simulink model "gm_ZynqBF_2tx_fpga"  (R2018b)
settings: Solver=FixedStepDiscrete  StartTime=0.0  StopTime=10.0  FixedStep=(1/420e3)/128  RelTol=1e-3
undefined symbols (not defined in the file or in its folder): a, b, c
libraries: hdlsllib x873, simulink x349
(part 20 of 40)

== system gm_ZynqBF_2tx_fpga/channel_estimator/peakdetect_ch1/correlator1/rx_ram_q_instance39 ==
  i : Inport  OutDataTypeStr=fixdt(0, 6, 0)  PortDimensions=1  SampleTime=1.86011904761905e-08
  wdata : Inport  Port=2  OutDataTypeStr=fixdt(1, 16, 15)  PortDimensions=1  SampleTime=1.86011904761905e-08
  waddr : Inport  Port=3  OutDataTypeStr=fixdt(0, 9, 0)  PortDimensions=1  SampleTime=1.86011904761905e-08
  we : Inport  Port=4  OutDataTypeStr=fixdt(0, 64, 0)  PortDimensions=1  SampleTime=1.86011904761905e-08
  raddr : Inport  Port=5  OutDataTypeStr=fixdt(0, 10, 0)  PortDimensions=1  SampleTime=1.86011904761905e-08
  shift : Inport  Port=6  OutDataTypeStr=fixdt(0, 6, 0)  PortDimensions=1  SampleTime=1.86011904761905e-08
  Constant : Constant  OutDataTypeStr=fixdt(0, 1, 0)  SampleTime=-1
  Constant1 : Constant  OutDataTypeStr=fixdt(0, 1, 0)  SampleTime=-1
  Relational Operator : RelationalOperator  Operator=<  OutDataTypeStr=boolean  SampleTime=1.86011904761905e-08  RndMeth=Nearest
  Simple Dual Port RAM : hdlsllib/HDL RAMs/Simple Dual Port RAM  ram_size=9
      settings: SourceProductName=HDL Coder  SourceProductBaseCode=HD
  Sum : Sum  AccumDataTypeStr=fixdt(0, 11, 0)  OutDataTypeStr=fixdt(0, 9, 0)  SampleTime=1.86011904761905e-08
  Sum1 : Sum  AccumDataTypeStr=fixdt(0, 7, 0)  OutDataTypeStr=fixdt(0, 9, 0)  SampleTime=1.86011904761905e-08
  Switch : Switch  Criteria=u2 ~= 0  Threshold=double(0)  OutDataTypeStr=fixdt(0, 9, 0)  SampleTime=1.86011904761905e-08
  get_bit : Subsystem
  dout : Outport
  probe : Outport  Port=2
  wires:
  shift/1 -> Relational Operator/2
  raddr/1 -> Switch/3, Sum/2
  we/1 -> get_bit/1(u)
  waddr/1 -> Simple Dual Port RAM/2
  wdata/1 -> Simple Dual Port RAM/1
  i/1 -> Sum1/1, Relational Operator/1
  Constant/1 -> Sum/1
  Constant1/1 -> Sum1/2
  Relational Operator/1 -> Switch/2
  Simple Dual Port RAM/1 -> dout/1
  Sum/1 -> Switch/1
  Sum1/1 -> get_bit/2(ind)
  Switch/1 -> Simple Dual Port RAM/4, probe/1
  get_bit/1(y) -> Simple Dual Port RAM/3

== system gm_ZynqBF_2tx_fpga/channel_estimator/peakdetect_ch1/correlator1/rx_ram_q_instance4 ==
  i : Inport  OutDataTypeStr=fixdt(0, 6, 0)  PortDimensions=1  SampleTime=1.86011904761905e-08
  wdata : Inport  Port=2  OutDataTypeStr=fixdt(1, 16, 15)  PortDimensions=1  SampleTime=1.86011904761905e-08
  waddr : Inport  Port=3  OutDataTypeStr=fixdt(0, 9, 0)  PortDimensions=1  SampleTime=1.86011904761905e-08
  we : Inport  Port=4  OutDataTypeStr=fixdt(0, 64, 0)  PortDimensions=1  SampleTime=1.86011904761905e-08
  raddr : Inport  Port=5  OutDataTypeStr=fixdt(0, 10, 0)  PortDimensions=1  SampleTime=1.86011904761905e-08
  shift : Inport  Port=6  OutDataTypeStr=fixdt(0, 6, 0)  PortDimensions=1  SampleTime=1.86011904761905e-08
  Constant : Constant  OutDataTypeStr=fixdt(0, 1, 0)  SampleTime=-1
  Constant1 : Constant  OutDataTypeStr=fixdt(0, 1, 0)  SampleTime=-1
  Relational Operator : RelationalOperator  Operator=<  OutDataTypeStr=boolean  SampleTime=1.86011904761905e-08  RndMeth=Nearest
  Simple Dual Port RAM : hdlsllib/HDL RAMs/Simple Dual Port RAM  ram_size=9
      settings: SourceProductName=HDL Coder  SourceProductBaseCode=HD
  Sum : Sum  AccumDataTypeStr=fixdt(0, 11, 0)  OutDataTypeStr=fixdt(0, 9, 0)  SampleTime=1.86011904761905e-08
  Sum1 : Sum  AccumDataTypeStr=fixdt(0, 7, 0)  OutDataTypeStr=fixdt(0, 9, 0)  SampleTime=1.86011904761905e-08
  Switch : Switch  Criteria=u2 ~= 0  Threshold=double(0)  OutDataTypeStr=fixdt(0, 9, 0)  SampleTime=1.86011904761905e-08
  get_bit : Subsystem
  dout : Outport
  probe : Outport  Port=2
  wires:
  shift/1 -> Relational Operator/2
  raddr/1 -> Switch/3, Sum/2
  we/1 -> get_bit/1(u)
  waddr/1 -> Simple Dual Port RAM/2
  wdata/1 -> Simple Dual Port RAM/1
  i/1 -> Sum1/1, Relational Operator/1
  Constant/1 -> Sum/1
  Constant1/1 -> Sum1/2
  Relational Operator/1 -> Switch/2
  Simple Dual Port RAM/1 -> dout/1
  Sum/1 -> Switch/1
  Sum1/1 -> get_bit/2(ind)
  Switch/1 -> Simple Dual Port RAM/4, probe/1
  get_bit/1(y) -> Simple Dual Port RAM/3

== system gm_ZynqBF_2tx_fpga/channel_estimator/peakdetect_ch1/correlator1/rx_ram_q_instance40 ==
  i : Inport  OutDataTypeStr=fixdt(0, 6, 0)  PortDimensions=1  SampleTime=1.86011904761905e-08
  wdata : Inport  Port=2  OutDataTypeStr=fixdt(1, 16, 15)  PortDimensions=1  SampleTime=1.86011904761905e-08
  waddr : Inport  Port=3  OutDataTypeStr=fixdt(0, 9, 0)  PortDimensions=1  SampleTime=1.86011904761905e-08
  we : Inport  Port=4  OutDataTypeStr=fixdt(0, 64, 0)  PortDimensions=1  SampleTime=1.86011904761905e-08
  raddr : Inport  Port=5  OutDataTypeStr=fixdt(0, 10, 0)  PortDimensions=1  SampleTime=1.86011904761905e-08
  shift : Inport  Port=6  OutDataTypeStr=fixdt(0, 6, 0)  PortDimensions=1  SampleTime=1.86011904761905e-08
  Constant : Constant  OutDataTypeStr=fixdt(0, 1, 0)  SampleTime=-1
  Constant1 : Constant  OutDataTypeStr=fixdt(0, 1, 0)  SampleTime=-1
  Relational Operator : RelationalOperator  Operator=<  OutDataTypeStr=boolean  SampleTime=1.86011904761905e-08  RndMeth=Nearest
  Simple Dual Port RAM : hdlsllib/HDL RAMs/Simple Dual Port RAM  ram_size=9
      settings: SourceProductName=HDL Coder  SourceProductBaseCode=HD
  Sum : Sum  AccumDataTypeStr=fixdt(0, 11, 0)  OutDataTypeStr=fixdt(0, 9, 0)  SampleTime=1.86011904761905e-08
  Sum1 : Sum  AccumDataTypeStr=fixdt(0, 7, 0)  OutDataTypeStr=fixdt(0, 9, 0)  SampleTime=1.86011904761905e-08
  Switch : Switch  Criteria=u2 ~= 0  Threshold=double(0)  OutDataTypeStr=fixdt(0, 9, 0)  SampleTime=1.86011904761905e-08
  get_bit : Subsystem
  dout : Outport
  probe : Outport  Port=2
  wires:
  shift/1 -> Relational Operator/2
  raddr/1 -> Switch/3, Sum/2
  we/1 -> get_bit/1(u)
  waddr/1 -> Simple Dual Port RAM/2
  wdata/1 -> Simple Dual Port RAM/1
  i/1 -> Sum1/1, Relational Operator/1
  Constant/1 -> Sum/1
  Constant1/1 -> Sum1/2
  Relational Operator/1 -> Switch/2
  Simple Dual Port RAM/1 -> dout/1
  Sum/1 -> Switch/1
  Sum1/1 -> get_bit/2(ind)
  Switch/1 -> Simple Dual Port RAM/4, probe/1
  get_bit/1(y) -> Simple Dual Port RAM/3

== system gm_ZynqBF_2tx_fpga/channel_estimator/peakdetect_ch1/correlator1/rx_ram_q_instance41 ==
  i : Inport  OutDataTypeStr=fixdt(0, 6, 0)  PortDimensions=1  SampleTime=1.86011904761905e-08
  wdata : Inport  Port=2  OutDataTypeStr=fixdt(1, 16, 15)  PortDimensions=1  SampleTime=1.86011904761905e-08
  waddr : Inport  Port=3  OutDataTypeStr=fixdt(0, 9, 0)  PortDimensions=1  SampleTime=1.86011904761905e-08
  we : Inport  Port=4  OutDataTypeStr=fixdt(0, 64, 0)  PortDimensions=1  SampleTime=1.86011904761905e-08
  raddr : Inport  Port=5  OutDataTypeStr=fixdt(0, 10, 0)  PortDimensions=1  SampleTime=1.86011904761905e-08
  shift : Inport  Port=6  OutDataTypeStr=fixdt(0, 6, 0)  PortDimensions=1  SampleTime=1.86011904761905e-08
  Constant : Constant  OutDataTypeStr=fixdt(0, 1, 0)  SampleTime=-1
  Constant1 : Constant  OutDataTypeStr=fixdt(0, 1, 0)  SampleTime=-1
  Relational Operator : RelationalOperator  Operator=<  OutDataTypeStr=boolean  SampleTime=1.86011904761905e-08  RndMeth=Nearest
  Simple Dual Port RAM : hdlsllib/HDL RAMs/Simple Dual Port RAM  ram_size=9
      settings: SourceProductName=HDL Coder  SourceProductBaseCode=HD
  Sum : Sum  AccumDataTypeStr=fixdt(0, 11, 0)  OutDataTypeStr=fixdt(0, 9, 0)  SampleTime=1.86011904761905e-08
  Sum1 : Sum  AccumDataTypeStr=fixdt(0, 7, 0)  OutDataTypeStr=fixdt(0, 9, 0)  SampleTime=1.86011904761905e-08
  Switch : Switch  Criteria=u2 ~= 0  Threshold=double(0)  OutDataTypeStr=fixdt(0, 9, 0)  SampleTime=1.86011904761905e-08
  get_bit : Subsystem
  dout : Outport
  probe : Outport  Port=2
  wires:
  shift/1 -> Relational Operator/2
  raddr/1 -> Switch/3, Sum/2
  we/1 -> get_bit/1(u)
  waddr/1 -> Simple Dual Port RAM/2
  wdata/1 -> Simple Dual Port RAM/1
  i/1 -> Sum1/1, Relational Operator/1
  Constant/1 -> Sum/1
  Constant1/1 -> Sum1/2
  Relational Operator/1 -> Switch/2
  Simple Dual Port RAM/1 -> dout/1
  Sum/1 -> Switch/1
  Sum1/1 -> get_bit/2(ind)
  Switch/1 -> Simple Dual Port RAM/4, probe/1
  get_bit/1(y) -> Simple Dual Port RAM/3

== system gm_ZynqBF_2tx_fpga/channel_estimator/peakdetect_ch1/correlator1/rx_ram_q_instance42 ==
  i : Inport  OutDataTypeStr=fixdt(0, 6, 0)  PortDimensions=1  SampleTime=1.86011904761905e-08
  wdata : Inport  Port=2  OutDataTypeStr=fixdt(1, 16, 15)  PortDimensions=1  SampleTime=1.86011904761905e-08
  waddr : Inport  Port=3  OutDataTypeStr=fixdt(0, 9, 0)  PortDimensions=1  SampleTime=1.86011904761905e-08
  we : Inport  Port=4  OutDataTypeStr=fixdt(0, 64, 0)  PortDimensions=1  SampleTime=1.86011904761905e-08
  raddr : Inport  Port=5  OutDataTypeStr=fixdt(0, 10, 0)  PortDimensions=1  SampleTime=1.86011904761905e-08
  shift : Inport  Port=6  OutDataTypeStr=fixdt(0, 6, 0)  PortDimensions=1  SampleTime=1.86011904761905e-08
  Constant : Constant  OutDataTypeStr=fixdt(0, 1, 0)  SampleTime=-1
  Constant1 : Constant  OutDataTypeStr=fixdt(0, 1, 0)  SampleTime=-1
  Relational Operator : RelationalOperator  Operator=<  OutDataTypeStr=boolean  SampleTime=1.86011904761905e-08  RndMeth=Nearest
  Simple Dual Port RAM : hdlsllib/HDL RAMs/Simple Dual Port RAM  ram_size=9
      settings: SourceProductName=HDL Coder  SourceProductBaseCode=HD
  Sum : Sum  AccumDataTypeStr=fixdt(0, 11, 0)  OutDataTypeStr=fixdt(0, 9, 0)  SampleTime=1.86011904761905e-08
  Sum1 : Sum  AccumDataTypeStr=fixdt(0, 7, 0)  OutDataTypeStr=fixdt(0, 9, 0)  SampleTime=1.86011904761905e-08
  Switch : Switch  Criteria=u2 ~= 0  Threshold=double(0)  OutDataTypeStr=fixdt(0, 9, 0)  SampleTime=1.86011904761905e-08
  get_bit : Subsystem
  dout : Outport
  probe : Outport  Port=2
  wires:
  shift/1 -> Relational Operator/2
  raddr/1 -> Switch/3, Sum/2
  we/1 -> get_bit/1(u)
  waddr/1 -> Simple Dual Port RAM/2
  wdata/1 -> Simple Dual Port RAM/1
  i/1 -> Sum1/1, Relational Operator/1
  Constant/1 -> Sum/1
  Constant1/1 -> Sum1/2
  Relational Operator/1 -> Switch/2
  Simple Dual Port RAM/1 -> dout/1
  Sum/1 -> Switch/1
  Sum1/1 -> get_bit/2(ind)
  Switch/1 -> Simple Dual Port RAM/4, probe/1
  get_bit/1(y) -> Simple Dual Port RAM/3

== system gm_ZynqBF_2tx_fpga/channel_estimator/peakdetect_ch1/correlator1/rx_ram_q_instance43 ==
  i : Inport  OutDataTypeStr=fixdt(0, 6, 0)  PortDimensions=1  SampleTime=1.86011904761905e-08
  wdata : Inport  Port=2  OutDataTypeStr=fixdt(1, 16, 15)  PortDimensions=1  SampleTime=1.86011904761905e-08
  waddr : Inport  Port=3  OutDataTypeStr=fixdt(0, 9, 0)  PortDimensions=1  SampleTime=1.86011904761905e-08
  we : Inport  Port=4  OutDataTypeStr=fixdt(0, 64, 0)  PortDimensions=1  SampleTime=1.86011904761905e-08
  raddr : Inport  Port=5  OutDataTypeStr=fixdt(0, 10, 0)  PortDimensions=1  SampleTime=1.86011904761905e-08
  shift : Inport  Port=6  OutDataTypeStr=fixdt(0, 6, 0)  PortDimensions=1  SampleTime=1.86011904761905e-08
  Constant : Constant  OutDataTypeStr=fixdt(0, 1, 0)  SampleTime=-1
  Constant1 : Constant  OutDataTypeStr=fixdt(0, 1, 0)  SampleTime=-1
  Relational Operator : RelationalOperator  Operator=<  OutDataTypeStr=boolean  SampleTime=1.86011904761905e-08  RndMeth=Nearest
  Simple Dual Port RAM : hdlsllib/HDL RAMs/Simple Dual Port RAM  ram_size=9
      settings: SourceProductName=HDL Coder  SourceProductBaseCode=HD
  Sum : Sum  AccumDataTypeStr=fixdt(0, 11, 0)  OutDataTypeStr=fixdt(0, 9, 0)  SampleTime=1.86011904761905e-08
  Sum1 : Sum  AccumDataTypeStr=fixdt(0, 7, 0)  OutDataTypeStr=fixdt(0, 9, 0)  SampleTime=1.86011904761905e-08
  Switch : Switch  Criteria=u2 ~= 0  Threshold=double(0)  OutDataTypeStr=fixdt(0, 9, 0)  SampleTime=1.86011904761905e-08
  get_bit : Subsystem
  dout : Outport
  probe : Outport  Port=2
  wires:
  shift/1 -> Relational Operator/2
  raddr/1 -> Switch/3, Sum/2
  we/1 -> get_bit/1(u)
  waddr/1 -> Simple Dual Port RAM/2
  wdata/1 -> Simple Dual Port RAM/1
  i/1 -> Sum1/1, Relational Operator/1
  Constant/1 -> Sum/1
  Constant1/1 -> Sum1/2
  Relational Operator/1 -> Switch/2
  Simple Dual Port RAM/1 -> dout/1
  Sum/1 -> Switch/1
  Sum1/1 -> get_bit/2(ind)
  Switch/1 -> Simple Dual Port RAM/4, probe/1
  get_bit/1(y) -> Simple Dual Port RAM/3

== system gm_ZynqBF_2tx_fpga/channel_estimator/peakdetect_ch1/correlator1/rx_ram_q_instance44 ==
  i : Inport  OutDataTypeStr=fixdt(0, 6, 0)  PortDimensions=1  SampleTime=1.86011904761905e-08
  wdata : Inport  Port=2  OutDataTypeStr=fixdt(1, 16, 15)  PortDimensions=1  SampleTime=1.86011904761905e-08
  waddr : Inport  Port=3  OutDataTypeStr=fixdt(0, 9, 0)  PortDimensions=1  SampleTime=1.86011904761905e-08
  we : Inport  Port=4  OutDataTypeStr=fixdt(0, 64, 0)  PortDimensions=1  SampleTime=1.86011904761905e-08
  raddr : Inport  Port=5  OutDataTypeStr=fixdt(0, 10, 0)  PortDimensions=1  SampleTime=1.86011904761905e-08
  shift : Inport  Port=6  OutDataTypeStr=fixdt(0, 6, 0)  PortDimensions=1  SampleTime=1.86011904761905e-08
  Constant : Constant  OutDataTypeStr=fixdt(0, 1, 0)  SampleTime=-1
  Constant1 : Constant  OutDataTypeStr=fixdt(0, 1, 0)  SampleTime=-1
  Relational Operator : RelationalOperator  Operator=<  OutDataTypeStr=boolean  SampleTime=1.86011904761905e-08  RndMeth=Nearest
  Simple Dual Port RAM : hdlsllib/HDL RAMs/Simple Dual Port RAM  ram_size=9
      settings: SourceProductName=HDL Coder  SourceProductBaseCode=HD
  Sum : Sum  AccumDataTypeStr=fixdt(0, 11, 0)  OutDataTypeStr=fixdt(0, 9, 0)  SampleTime=1.86011904761905e-08
  Sum1 : Sum  AccumDataTypeStr=fixdt(0, 7, 0)  OutDataTypeStr=fixdt(0, 9, 0)  SampleTime=1.86011904761905e-08
  Switch : Switch  Criteria=u2 ~= 0  Threshold=double(0)  OutDataTypeStr=fixdt(0, 9, 0)  SampleTime=1.86011904761905e-08
  get_bit : Subsystem
  dout : Outport
  probe : Outport  Port=2
  wires:
  shift/1 -> Relational Operator/2
  raddr/1 -> Switch/3, Sum/2
  we/1 -> get_bit/1(u)
  waddr/1 -> Simple Dual Port RAM/2
  wdata/1 -> Simple Dual Port RAM/1
  i/1 -> Sum1/1, Relational Operator/1
  Constant/1 -> Sum/1
  Constant1/1 -> Sum1/2
  Relational Operator/1 -> Switch/2
  Simple Dual Port RAM/1 -> dout/1
  Sum/1 -> Switch/1
  Sum1/1 -> get_bit/2(ind)
  Switch/1 -> Simple Dual Port RAM/4, probe/1
  get_bit/1(y) -> Simple Dual Port RAM/3

== system gm_ZynqBF_2tx_fpga/channel_estimator/peakdetect_ch1/correlator1/rx_ram_q_instance45 ==
  i : Inport  OutDataTypeStr=fixdt(0, 6, 0)  PortDimensions=1  SampleTime=1.86011904761905e-08
  wdata : Inport  Port=2  OutDataTypeStr=fixdt(1, 16, 15)  PortDimensions=1  SampleTime=1.86011904761905e-08
  waddr : Inport  Port=3  OutDataTypeStr=fixdt(0, 9, 0)  PortDimensions=1  SampleTime=1.86011904761905e-08
  we : Inport  Port=4  OutDataTypeStr=fixdt(0, 64, 0)  PortDimensions=1  SampleTime=1.86011904761905e-08
  raddr : Inport  Port=5  OutDataTypeStr=fixdt(0, 10, 0)  PortDimensions=1  SampleTime=1.86011904761905e-08
  shift : Inport  Port=6  OutDataTypeStr=fixdt(0, 6, 0)  PortDimensions=1  SampleTime=1.86011904761905e-08
  Constant : Constant  OutDataTypeStr=fixdt(0, 1, 0)  SampleTime=-1
  Constant1 : Constant  OutDataTypeStr=fixdt(0, 1, 0)  SampleTime=-1
  Relational Operator : RelationalOperator  Operator=<  OutDataTypeStr=boolean  SampleTime=1.86011904761905e-08  RndMeth=Nearest
  Simple Dual Port RAM : hdlsllib/HDL RAMs/Simple Dual Port RAM  ram_size=9
      settings: SourceProductName=HDL Coder  SourceProductBaseCode=HD
  Sum : Sum  AccumDataTypeStr=fixdt(0, 11, 0)  OutDataTypeStr=fixdt(0, 9, 0)  SampleTime=1.86011904761905e-08
  Sum1 : Sum  AccumDataTypeStr=fixdt(0, 7, 0)  OutDataTypeStr=fixdt(0, 9, 0)  SampleTime=1.86011904761905e-08
  Switch : Switch  Criteria=u2 ~= 0  Threshold=double(0)  OutDataTypeStr=fixdt(0, 9, 0)  SampleTime=1.86011904761905e-08
  get_bit : Subsystem
  dout : Outport
  probe : Outport  Port=2
  wires:
  shift/1 -> Relational Operator/2
  raddr/1 -> Switch/3, Sum/2
  we/1 -> get_bit/1(u)
  waddr/1 -> Simple Dual Port RAM/2
  wdata/1 -> Simple Dual Port RAM/1
  i/1 -> Sum1/1, Relational Operator/1
  Constant/1 -> Sum/1
  Constant1/1 -> Sum1/2
  Relational Operator/1 -> Switch/2
  Simple Dual Port RAM/1 -> dout/1
  Sum/1 -> Switch/1
  Sum1/1 -> get_bit/2(ind)
  Switch/1 -> Simple Dual Port RAM/4, probe/1
  get_bit/1(y) -> Simple Dual Port RAM/3

== system gm_ZynqBF_2tx_fpga/channel_estimator/peakdetect_ch1/correlator1/rx_ram_q_instance46 ==
  i : Inport  OutDataTypeStr=fixdt(0, 6, 0)  PortDimensions=1  SampleTime=1.86011904761905e-08
  wdata : Inport  Port=2  OutDataTypeStr=fixdt(1, 16, 15)  PortDimensions=1  SampleTime=1.86011904761905e-08
  waddr : Inport  Port=3  OutDataTypeStr=fixdt(0, 9, 0)  PortDimensions=1  SampleTime=1.86011904761905e-08
  we : Inport  Port=4  OutDataTypeStr=fixdt(0, 64, 0)  PortDimensions=1  SampleTime=1.86011904761905e-08
  raddr : Inport  Port=5  OutDataTypeStr=fixdt(0, 10, 0)  PortDimensions=1  SampleTime=1.86011904761905e-08
  shift : Inport  Port=6  OutDataTypeStr=fixdt(0, 6, 0)  PortDimensions=1  SampleTime=1.86011904761905e-08
  Constant : Constant  OutDataTypeStr=fixdt(0, 1, 0)  SampleTime=-1
  Constant1 : Constant  OutDataTypeStr=fixdt(0, 1, 0)  SampleTime=-1
  Relational Operator : RelationalOperator  Operator=<  OutDataTypeStr=boolean  SampleTime=1.86011904761905e-08  RndMeth=Nearest
  Simple Dual Port RAM : hdlsllib/HDL RAMs/Simple Dual Port RAM  ram_size=9
      settings: SourceProductName=HDL Coder  SourceProductBaseCode=HD
  Sum : Sum  AccumDataTypeStr=fixdt(0, 11, 0)  OutDataTypeStr=fixdt(0, 9, 0)  SampleTime=1.86011904761905e-08
  Sum1 : Sum  AccumDataTypeStr=fixdt(0, 7, 0)  OutDataTypeStr=fixdt(0, 9, 0)  SampleTime=1.86011904761905e-08
  Switch : Switch  Criteria=u2 ~= 0  Threshold=double(0)  OutDataTypeStr=fixdt(0, 9, 0)  SampleTime=1.86011904761905e-08
  get_bit : Subsystem
  dout : Outport
  probe : Outport  Port=2
  wires:
  shift/1 -> Relational Operator/2
  raddr/1 -> Switch/3, Sum/2
  we/1 -> get_bit/1(u)
  waddr/1 -> Simple Dual Port RAM/2
  wdata/1 -> Simple Dual Port RAM/1
  i/1 -> Sum1/1, Relational Operator/1
  Constant/1 -> Sum/1
  Constant1/1 -> Sum1/2
  Relational Operator/1 -> Switch/2
  Simple Dual Port RAM/1 -> dout/1
  Sum/1 -> Switch/1
  Sum1/1 -> get_bit/2(ind)
  Switch/1 -> Simple Dual Port RAM/4, probe/1
  get_bit/1(y) -> Simple Dual Port RAM/3

== system gm_ZynqBF_2tx_fpga/channel_estimator/peakdetect_ch1/correlator1/rx_ram_q_instance47 ==
  i : Inport  OutDataTypeStr=fixdt(0, 6, 0)  PortDimensions=1  SampleTime=1.86011904761905e-08
  wdata : Inport  Port=2  OutDataTypeStr=fixdt(1, 16, 15)  PortDimensions=1  SampleTime=1.86011904761905e-08
  waddr : Inport  Port=3  OutDataTypeStr=fixdt(0, 9, 0)  PortDimensions=1  SampleTime=1.86011904761905e-08
  we : Inport  Port=4  OutDataTypeStr=fixdt(0, 64, 0)  PortDimensions=1  SampleTime=1.86011904761905e-08
  raddr : Inport  Port=5  OutDataTypeStr=fixdt(0, 10, 0)  PortDimensions=1  SampleTime=1.86011904761905e-08
  shift : Inport  Port=6  OutDataTypeStr=fixdt(0, 6, 0)  PortDimensions=1  SampleTime=1.86011904761905e-08
  Constant : Constant  OutDataTypeStr=fixdt(0, 1, 0)  SampleTime=-1
  Constant1 : Constant  OutDataTypeStr=fixdt(0, 1, 0)  SampleTime=-1
  Relational Operator : RelationalOperator  Operator=<  OutDataTypeStr=boolean  SampleTime=1.86011904761905e-08  RndMeth=Nearest
  Simple Dual Port RAM : hdlsllib/HDL RAMs/Simple Dual Port RAM  ram_size=9
      settings: SourceProductName=HDL Coder  SourceProductBaseCode=HD
  Sum : Sum  AccumDataTypeStr=fixdt(0, 11, 0)  OutDataTypeStr=fixdt(0, 9, 0)  SampleTime=1.86011904761905e-08
  Sum1 : Sum  AccumDataTypeStr=fixdt(0, 7, 0)  OutDataTypeStr=fixdt(0, 9, 0)  SampleTime=1.86011904761905e-08
  Switch : Switch  Criteria=u2 ~= 0  Threshold=double(0)  OutDataTypeStr=fixdt(0, 9, 0)  SampleTime=1.86011904761905e-08
  get_bit : Subsystem
  dout : Outport
  probe : Outport  Port=2
  wires:
  shift/1 -> Relational Operator/2
  raddr/1 -> Switch/3, Sum/2
  we/1 -> get_bit/1(u)
  waddr/1 -> Simple Dual Port RAM/2
  wdata/1 -> Simple Dual Port RAM/1
  i/1 -> Sum1/1, Relational Operator/1
  Constant/1 -> Sum/1
  Constant1/1 -> Sum1/2
  Relational Operator/1 -> Switch/2
  Simple Dual Port RAM/1 -> dout/1
  Sum/1 -> Switch/1
  Sum1/1 -> get_bit/2(ind)
  Switch/1 -> Simple Dual Port RAM/4, probe/1
  get_bit/1(y) -> Simple Dual Port RAM/3

== system gm_ZynqBF_2tx_fpga/channel_estimator/peakdetect_ch1/correlator1/rx_ram_q_instance48 ==
  i : Inport  OutDataTypeStr=fixdt(0, 6, 0)  PortDimensions=1  SampleTime=1.86011904761905e-08
  wdata : Inport  Port=2  OutDataTypeStr=fixdt(1, 16, 15)  PortDimensions=1  SampleTime=1.86011904761905e-08
  waddr : Inport  Port=3  OutDataTypeStr=fixdt(0, 9, 0)  PortDimensions=1  SampleTime=1.86011904761905e-08
  we : Inport  Port=4  OutDataTypeStr=fixdt(0, 64, 0)  PortDimensions=1  SampleTime=1.86011904761905e-08
  raddr : Inport  Port=5  OutDataTypeStr=fixdt(0, 10, 0)  PortDimensions=1  SampleTime=1.86011904761905e-08
  shift : Inport  Port=6  OutDataTypeStr=fixdt(0, 6, 0)  PortDimensions=1  SampleTime=1.86011904761905e-08
  Constant : Constant  OutDataTypeStr=fixdt(0, 1, 0)  SampleTime=-1
  Constant1 : Constant  OutDataTypeStr=fixdt(0, 1, 0)  SampleTime=-1
  Relational Operator : RelationalOperator  Operator=<  OutDataTypeStr=boolean  SampleTime=1.86011904761905e-08  RndMeth=Nearest
  Simple Dual Port RAM : hdlsllib/HDL RAMs/Simple Dual Port RAM  ram_size=9
      settings: SourceProductName=HDL Coder  SourceProductBaseCode=HD
  Sum : Sum  AccumDataTypeStr=fixdt(0, 11, 0)  OutDataTypeStr=fixdt(0, 9, 0)  SampleTime=1.86011904761905e-08
  Sum1 : Sum  AccumDataTypeStr=fixdt(0, 7, 0)  OutDataTypeStr=fixdt(0, 9, 0)  SampleTime=1.86011904761905e-08
  Switch : Switch  Criteria=u2 ~= 0  Threshold=double(0)  OutDataTypeStr=fixdt(0, 9, 0)  SampleTime=1.86011904761905e-08
  get_bit : Subsystem
  dout : Outport
  probe : Outport  Port=2
  wires:
  shift/1 -> Relational Operator/2
  raddr/1 -> Switch/3, Sum/2
  we/1 -> get_bit/1(u)
  waddr/1 -> Simple Dual Port RAM/2
  wdata/1 -> Simple Dual Port RAM/1
  i/1 -> Sum1/1, Relational Operator/1
  Constant/1 -> Sum/1
  Constant1/1 -> Sum1/2
  Relational Operator/1 -> Switch/2
  Simple Dual Port RAM/1 -> dout/1
  Sum/1 -> Switch/1
  Sum1/1 -> get_bit/2(ind)
  Switch/1 -> Simple Dual Port RAM/4, probe/1
  get_bit/1(y) -> Simple Dual Port RAM/3

== system gm_ZynqBF_2tx_fpga/channel_estimator/peakdetect_ch1/correlator1/rx_ram_q_instance49 ==
  i : Inport  OutDataTypeStr=fixdt(0, 6, 0)  PortDimensions=1  SampleTime=1.86011904761905e-08
  wdata : Inport  Port=2  OutDataTypeStr=fixdt(1, 16, 15)  PortDimensions=1  SampleTime=1.86011904761905e-08
  waddr : Inport  Port=3  OutDataTypeStr=fixdt(0, 9, 0)  PortDimensions=1  SampleTime=1.86011904761905e-08
  we : Inport  Port=4  OutDataTypeStr=fixdt(0, 64, 0)  PortDimensions=1  SampleTime=1.86011904761905e-08
  raddr : Inport  Port=5  OutDataTypeStr=fixdt(0, 10, 0)  PortDimensions=1  SampleTime=1.86011904761905e-08
  shift : Inport  Port=6  OutDataTypeStr=fixdt(0, 6, 0)  PortDimensions=1  SampleTime=1.86011904761905e-08
  Constant : Constant  OutDataTypeStr=fixdt(0, 1, 0)  SampleTime=-1
  Constant1 : Constant  OutDataTypeStr=fixdt(0, 1, 0)  SampleTime=-1
  Relational Operator : RelationalOperator  Operator=<  OutDataTypeStr=boolean  SampleTime=1.86011904761905e-08  RndMeth=Nearest
  Simple Dual Port RAM : hdlsllib/HDL RAMs/Simple Dual Port RAM  ram_size=9
      settings: SourceProductName=HDL Coder  SourceProductBaseCode=HD
  Sum : Sum  AccumDataTypeStr=fixdt(0, 11, 0)  OutDataTypeStr=fixdt(0, 9, 0)  SampleTime=1.86011904761905e-08
  Sum1 : Sum  AccumDataTypeStr=fixdt(0, 7, 0)  OutDataTypeStr=fixdt(0, 9, 0)  SampleTime=1.86011904761905e-08
  Switch : Switch  Criteria=u2 ~= 0  Threshold=double(0)  OutDataTypeStr=fixdt(0, 9, 0)  SampleTime=1.86011904761905e-08
  get_bit : Subsystem
  dout : Outport
  probe : Outport  Port=2
  wires:
  shift/1 -> Relational Operator/2
  raddr/1 -> Switch/3, Sum/2
  we/1 -> get_bit/1(u)
  waddr/1 -> Simple Dual Port RAM/2
  wdata/1 -> Simple Dual Port RAM/1
  i/1 -> Sum1/1, Relational Operator/1
  Constant/1 -> Sum/1
  Constant1/1 -> Sum1/2
  Relational Operator/1 -> Switch/2
  Simple Dual Port RAM/1 -> dout/1
  Sum/1 -> Switch/1
  Sum1/1 -> get_bit/2(ind)
  Switch/1 -> Simple Dual Port RAM/4, probe/1
  get_bit/1(y) -> Simple Dual Port RAM/3

== system gm_ZynqBF_2tx_fpga/channel_estimator/peakdetect_ch1/correlator1/rx_ram_q_instance5 ==
  i : Inport  OutDataTypeStr=fixdt(0, 6, 0)  PortDimensions=1  SampleTime=1.86011904761905e-08
  wdata : Inport  Port=2  OutDataTypeStr=fixdt(1, 16, 15)  PortDimensions=1  SampleTime=1.86011904761905e-08
  waddr : Inport  Port=3  OutDataTypeStr=fixdt(0, 9, 0)  PortDimensions=1  SampleTime=1.86011904761905e-08
  we : Inport  Port=4  OutDataTypeStr=fixdt(0, 64, 0)  PortDimensions=1  SampleTime=1.86011904761905e-08
  raddr : Inport  Port=5  OutDataTypeStr=fixdt(0, 10, 0)  PortDimensions=1  SampleTime=1.86011904761905e-08
  shift : Inport  Port=6  OutDataTypeStr=fixdt(0, 6, 0)  PortDimensions=1  SampleTime=1.86011904761905e-08
  Constant : Constant  OutDataTypeStr=fixdt(0, 1, 0)  SampleTime=-1
  Constant1 : Constant  OutDataTypeStr=fixdt(0, 1, 0)  SampleTime=-1
  Relational Operator : RelationalOperator  Operator=<  OutDataTypeStr=boolean  SampleTime=1.86011904761905e-08  RndMeth=Nearest
  Simple Dual Port RAM : hdlsllib/HDL RAMs/Simple Dual Port RAM  ram_size=9
      settings: SourceProductName=HDL Coder  SourceProductBaseCode=HD
  Sum : Sum  AccumDataTypeStr=fixdt(0, 11, 0)  OutDataTypeStr=fixdt(0, 9, 0)  SampleTime=1.86011904761905e-08
  Sum1 : Sum  AccumDataTypeStr=fixdt(0, 7, 0)  OutDataTypeStr=fixdt(0, 9, 0)  SampleTime=1.86011904761905e-08
  Switch : Switch  Criteria=u2 ~= 0  Threshold=double(0)  OutDataTypeStr=fixdt(0, 9, 0)  SampleTime=1.86011904761905e-08
  get_bit : Subsystem
  dout : Outport
  probe : Outport  Port=2
  wires:
  shift/1 -> Relational Operator/2
  raddr/1 -> Switch/3, Sum/2
  we/1 -> get_bit/1(u)
  waddr/1 -> Simple Dual Port RAM/2
  wdata/1 -> Simple Dual Port RAM/1
  i/1 -> Sum1/1, Relational Operator/1
  Constant/1 -> Sum/1
  Constant1/1 -> Sum1/2
  Relational Operator/1 -> Switch/2
  Simple Dual Port RAM/1 -> dout/1
  Sum/1 -> Switch/1
  Sum1/1 -> get_bit/2(ind)
  Switch/1 -> Simple Dual Port RAM/4, probe/1
  get_bit/1(y) -> Simple Dual Port RAM/3

== system gm_ZynqBF_2tx_fpga/channel_estimator/peakdetect_ch1/correlator1/rx_ram_q_instance50 ==
  i : Inport  OutDataTypeStr=fixdt(0, 6, 0)  PortDimensions=1  SampleTime=1.86011904761905e-08
  wdata : Inport  Port=2  OutDataTypeStr=fixdt(1, 16, 15)  PortDimensions=1  SampleTime=1.86011904761905e-08
  waddr : Inport  Port=3  OutDataTypeStr=fixdt(0, 9, 0)  PortDimensions=1  SampleTime=1.86011904761905e-08
  we : Inport  Port=4  OutDataTypeStr=fixdt(0, 64, 0)  PortDimensions=1  SampleTime=1.86011904761905e-08
  raddr : Inport  Port=5  OutDataTypeStr=fixdt(0, 10, 0)  PortDimensions=1  SampleTime=1.86011904761905e-08
  shift : Inport  Port=6  OutDataTypeStr=fixdt(0, 6, 0)  PortDimensions=1  SampleTime=1.86011904761905e-08
  Constant : Constant  OutDataTypeStr=fixdt(0, 1, 0)  SampleTime=-1
  Constant1 : Constant  OutDataTypeStr=fixdt(0, 1, 0)  SampleTime=-1
  Relational Operator : RelationalOperator  Operator=<  OutDataTypeStr=boolean  SampleTime=1.86011904761905e-08  RndMeth=Nearest
  Simple Dual Port RAM : hdlsllib/HDL RAMs/Simple Dual Port RAM  ram_size=9
      settings: SourceProductName=HDL Coder  SourceProductBaseCode=HD
  Sum : Sum  AccumDataTypeStr=fixdt(0, 11, 0)  OutDataTypeStr=fixdt(0, 9, 0)  SampleTime=1.86011904761905e-08
  Sum1 : Sum  AccumDataTypeStr=fixdt(0, 7, 0)  OutDataTypeStr=fixdt(0, 9, 0)  SampleTime=1.86011904761905e-08
  Switch : Switch  Criteria=u2 ~= 0  Threshold=double(0)  OutDataTypeStr=fixdt(0, 9, 0)  SampleTime=1.86011904761905e-08
  get_bit : Subsystem
  dout : Outport
  probe : Outport  Port=2
  wires:
  shift/1 -> Relational Operator/2
  raddr/1 -> Switch/3, Sum/2
  we/1 -> get_bit/1(u)
  waddr/1 -> Simple Dual Port RAM/2
  wdata/1 -> Simple Dual Port RAM/1
  i/1 -> Sum1/1, Relational Operator/1
  Constant/1 -> Sum/1
  Constant1/1 -> Sum1/2
  Relational Operator/1 -> Switch/2
  Simple Dual Port RAM/1 -> dout/1
  Sum/1 -> Switch/1
  Sum1/1 -> get_bit/2(ind)
  Switch/1 -> Simple Dual Port RAM/4, probe/1
  get_bit/1(y) -> Simple Dual Port RAM/3

== system gm_ZynqBF_2tx_fpga/channel_estimator/peakdetect_ch1/correlator1/rx_ram_q_instance51 ==
  i : Inport  OutDataTypeStr=fixdt(0, 6, 0)  PortDimensions=1  SampleTime=1.86011904761905e-08
  wdata : Inport  Port=2  OutDataTypeStr=fixdt(1, 16, 15)  PortDimensions=1  SampleTime=1.86011904761905e-08
  waddr : Inport  Port=3  OutDataTypeStr=fixdt(0, 9, 0)  PortDimensions=1  SampleTime=1.86011904761905e-08
  we : Inport  Port=4  OutDataTypeStr=fixdt(0, 64, 0)  PortDimensions=1  SampleTime=1.86011904761905e-08
  raddr : Inport  Port=5  OutDataTypeStr=fixdt(0, 10, 0)  PortDimensions=1  SampleTime=1.86011904761905e-08
  shift : Inport  Port=6  OutDataTypeStr=fixdt(0, 6, 0)  PortDimensions=1  SampleTime=1.86011904761905e-08
  Constant : Constant  OutDataTypeStr=fixdt(0, 1, 0)  SampleTime=-1
  Constant1 : Constant  OutDataTypeStr=fixdt(0, 1, 0)  SampleTime=-1
  Relational Operator : RelationalOperator  Operator=<  OutDataTypeStr=boolean  SampleTime=1.86011904761905e-08  RndMeth=Nearest
  Simple Dual Port RAM : hdlsllib/HDL RAMs/Simple Dual Port RAM  ram_size=9
      settings: SourceProductName=HDL Coder  SourceProductBaseCode=HD
  Sum : Sum  AccumDataTypeStr=fixdt(0, 11, 0)  OutDataTypeStr=fixdt(0, 9, 0)  SampleTime=1.86011904761905e-08
  Sum1 : Sum  AccumDataTypeStr=fixdt(0, 7, 0)  OutDataTypeStr=fixdt(0, 9, 0)  SampleTime=1.86011904761905e-08
  Switch : Switch  Criteria=u2 ~= 0  Threshold=double(0)  OutDataTypeStr=fixdt(0, 9, 0)  SampleTime=1.86011904761905e-08
  get_bit : Subsystem
  dout : Outport
  probe : Outport  Port=2
  wires:
  shift/1 -> Relational Operator/2
  raddr/1 -> Switch/3, Sum/2
  we/1 -> get_bit/1(u)
  waddr/1 -> Simple Dual Port RAM/2
  wdata/1 -> Simple Dual Port RAM/1
  i/1 -> Sum1/1, Relational Operator/1
  Constant/1 -> Sum/1
  Constant1/1 -> Sum1/2
  Relational Operator/1 -> Switch/2
  Simple Dual Port RAM/1 -> dout/1
  Sum/1 -> Switch/1
  Sum1/1 -> get_bit/2(ind)
  Switch/1 -> Simple Dual Port RAM/4, probe/1
  get_bit/1(y) -> Simple Dual Port RAM/3

== system gm_ZynqBF_2tx_fpga/channel_estimator/peakdetect_ch1/correlator1/rx_ram_q_instance52 ==
  i : Inport  OutDataTypeStr=fixdt(0, 6, 0)  PortDimensions=1  SampleTime=1.86011904761905e-08
  wdata : Inport  Port=2  OutDataTypeStr=fixdt(1, 16, 15)  PortDimensions=1  SampleTime=1.86011904761905e-08
  waddr : Inport  Port=3  OutDataTypeStr=fixdt(0, 9, 0)  PortDimensions=1  SampleTime=1.86011904761905e-08
  we : Inport  Port=4  OutDataTypeStr=fixdt(0, 64, 0)  PortDimensions=1  SampleTime=1.86011904761905e-08
  raddr : Inport  Port=5  OutDataTypeStr=fixdt(0, 10, 0)  PortDimensions=1  SampleTime=1.86011904761905e-08
  shift : Inport  Port=6  OutDataTypeStr=fixdt(0, 6, 0)  PortDimensions=1  SampleTime=1.86011904761905e-08
  Constant : Constant  OutDataTypeStr=fixdt(0, 1, 0)  SampleTime=-1
  Constant1 : Constant  OutDataTypeStr=fixdt(0, 1, 0)  SampleTime=-1
  Relational Operator : RelationalOperator  Operator=<  OutDataTypeStr=boolean  SampleTime=1.86011904761905e-08  RndMeth=Nearest
  Simple Dual Port RAM : hdlsllib/HDL RAMs/Simple Dual Port RAM  ram_size=9
      settings: SourceProductName=HDL Coder  SourceProductBaseCode=HD
  Sum : Sum  AccumDataTypeStr=fixdt(0, 11, 0)  OutDataTypeStr=fixdt(0, 9, 0)  SampleTime=1.86011904761905e-08
  Sum1 : Sum  AccumDataTypeStr=fixdt(0, 7, 0)  OutDataTypeStr=fixdt(0, 9, 0)  SampleTime=1.86011904761905e-08
  Switch : Switch  Criteria=u2 ~= 0  Threshold=double(0)  OutDataTypeStr=fixdt(0, 9, 0)  SampleTime=1.86011904761905e-08
  get_bit : Subsystem
  dout : Outport
  probe : Outport  Port=2
  wires:
  shift/1 -> Relational Operator/2
  raddr/1 -> Switch/3, Sum/2
  we/1 -> get_bit/1(u)
  waddr/1 -> Simple Dual Port RAM/2
  wdata/1 -> Simple Dual Port RAM/1
  i/1 -> Sum1/1, Relational Operator/1
  Constant/1 -> Sum/1
  Constant1/1 -> Sum1/2
  Relational Operator/1 -> Switch/2
  Simple Dual Port RAM/1 -> dout/1
  Sum/1 -> Switch/1
  Sum1/1 -> get_bit/2(ind)
  Switch/1 -> Simple Dual Port RAM/4, probe/1
  get_bit/1(y) -> Simple Dual Port RAM/3

== system gm_ZynqBF_2tx_fpga/channel_estimator/peakdetect_ch1/correlator1/rx_ram_q_instance53 ==
  i : Inport  OutDataTypeStr=fixdt(0, 6, 0)  PortDimensions=1  SampleTime=1.86011904761905e-08
  wdata : Inport  Port=2  OutDataTypeStr=fixdt(1, 16, 15)  PortDimensions=1  SampleTime=1.86011904761905e-08
  waddr : Inport  Port=3  OutDataTypeStr=fixdt(0, 9, 0)  PortDimensions=1  SampleTime=1.86011904761905e-08
  we : Inport  Port=4  OutDataTypeStr=fixdt(0, 64, 0)  PortDimensions=1  SampleTime=1.86011904761905e-08
  raddr : Inport  Port=5  OutDataTypeStr=fixdt(0, 10, 0)  PortDimensions=1  SampleTime=1.86011904761905e-08
  shift : Inport  Port=6  OutDataTypeStr=fixdt(0, 6, 0)  PortDimensions=1  SampleTime=1.86011904761905e-08
  Constant : Constant  OutDataTypeStr=fixdt(0, 1, 0)  SampleTime=-1
  Constant1 : Constant  OutDataTypeStr=fixdt(0, 1, 0)  SampleTime=-1
  Relational Operator : RelationalOperator  Operator=<  OutDataTypeStr=boolean  SampleTime=1.86011904761905e-08  RndMeth=Nearest
  Simple Dual Port RAM : hdlsllib/HDL RAMs/Simple Dual Port RAM  ram_size=9
      settings: SourceProductName=HDL Coder  SourceProductBaseCode=HD
  Sum : Sum  AccumDataTypeStr=fixdt(0, 11, 0)  OutDataTypeStr=fixdt(0, 9, 0)  SampleTime=1.86011904761905e-08
  Sum1 : Sum  AccumDataTypeStr=fixdt(0, 7, 0)  OutDataTypeStr=fixdt(0, 9, 0)  SampleTime=1.86011904761905e-08
  Switch : Switch  Criteria=u2 ~= 0  Threshold=double(0)  OutDataTypeStr=fixdt(0, 9, 0)  SampleTime=1.86011904761905e-08
  get_bit : Subsystem
  dout : Outport
  probe : Outport  Port=2
  wires:
  shift/1 -> Relational Operator/2
  raddr/1 -> Switch/3, Sum/2
  we/1 -> get_bit/1(u)
  waddr/1 -> Simple Dual Port RAM/2
  wdata/1 -> Simple Dual Port RAM/1
  i/1 -> Sum1/1, Relational Operator/1
  Constant/1 -> Sum/1
  Constant1/1 -> Sum1/2
  Relational Operator/1 -> Switch/2
  Simple Dual Port RAM/1 -> dout/1
  Sum/1 -> Switch/1
  Sum1/1 -> get_bit/2(ind)
  Switch/1 -> Simple Dual Port RAM/4, probe/1
  get_bit/1(y) -> Simple Dual Port RAM/3

== system gm_ZynqBF_2tx_fpga/channel_estimator/peakdetect_ch1/correlator1/rx_ram_q_instance54 ==
  i : Inport  OutDataTypeStr=fixdt(0, 6, 0)  PortDimensions=1  SampleTime=1.86011904761905e-08
  wdata : Inport  Port=2  OutDataTypeStr=fixdt(1, 16, 15)  PortDimensions=1  SampleTime=1.86011904761905e-08
  waddr : Inport  Port=3  OutDataTypeStr=fixdt(0, 9, 0)  PortDimensions=1  SampleTime=1.86011904761905e-08
  we : Inport  Port=4  OutDataTypeStr=fixdt(0, 64, 0)  PortDimensions=1  SampleTime=1.86011904761905e-08
  raddr : Inport  Port=5  OutDataTypeStr=fixdt(0, 10, 0)  PortDimensions=1  SampleTime=1.86011904761905e-08
  shift : Inport  Port=6  OutDataTypeStr=fixdt(0, 6, 0)  PortDimensions=1  SampleTime=1.86011904761905e-08
  Constant : Constant  OutDataTypeStr=fixdt(0, 1, 0)  SampleTime=-1
  Constant1 : Constant  OutDataTypeStr=fixdt(0, 1, 0)  SampleTime=-1
  Relational Operator : RelationalOperator  Operator=<  OutDataTypeStr=boolean  SampleTime=1.86011904761905e-08  RndMeth=Nearest
  Simple Dual Port RAM : hdlsllib/HDL RAMs/Simple Dual Port RAM  ram_size=9
      settings: SourceProductName=HDL Coder  SourceProductBaseCode=HD
  Sum : Sum  AccumDataTypeStr=fixdt(0, 11, 0)  OutDataTypeStr=fixdt(0, 9, 0)  SampleTime=1.86011904761905e-08
  Sum1 : Sum  AccumDataTypeStr=fixdt(0, 7, 0)  OutDataTypeStr=fixdt(0, 9, 0)  SampleTime=1.86011904761905e-08
  Switch : Switch  Criteria=u2 ~= 0  Threshold=double(0)  OutDataTypeStr=fixdt(0, 9, 0)  SampleTime=1.86011904761905e-08
  get_bit : Subsystem
  dout : Outport
  probe : Outport  Port=2
  wires:
  shift/1 -> Relational Operator/2
  raddr/1 -> Switch/3, Sum/2
  we/1 -> get_bit/1(u)
  waddr/1 -> Simple Dual Port RAM/2
  wdata/1 -> Simple Dual Port RAM/1
  i/1 -> Sum1/1, Relational Operator/1
  Constant/1 -> Sum/1
  Constant1/1 -> Sum1/2
  Relational Operator/1 -> Switch/2
  Simple Dual Port RAM/1 -> dout/1
  Sum/1 -> Switch/1
  Sum1/1 -> get_bit/2(ind)
  Switch/1 -> Simple Dual Port RAM/4, probe/1
  get_bit/1(y) -> Simple Dual Port RAM/3

== system gm_ZynqBF_2tx_fpga/channel_estimator/peakdetect_ch1/correlator1/rx_ram_q_instance55 ==
  i : Inport  OutDataTypeStr=fixdt(0, 6, 0)  PortDimensions=1  SampleTime=1.86011904761905e-08
  wdata : Inport  Port=2  OutDataTypeStr=fixdt(1, 16, 15)  PortDimensions=1  SampleTime=1.86011904761905e-08
  waddr : Inport  Port=3  OutDataTypeStr=fixdt(0, 9, 0)  PortDimensions=1  SampleTime=1.86011904761905e-08
  we : Inport  Port=4  OutDataTypeStr=fixdt(0, 64, 0)  PortDimensions=1  SampleTime=1.86011904761905e-08
  raddr : Inport  Port=5  OutDataTypeStr=fixdt(0, 10, 0)  PortDimensions=1  SampleTime=1.86011904761905e-08
  shift : Inport  Port=6  OutDataTypeStr=fixdt(0, 6, 0)  PortDimensions=1  SampleTime=1.86011904761905e-08
  Constant : Constant  OutDataTypeStr=fixdt(0, 1, 0)  SampleTime=-1
  Constant1 : Constant  OutDataTypeStr=fixdt(0, 1, 0)  SampleTime=-1
  Relational Operator : RelationalOperator  Operator=<  OutDataTypeStr=boolean  SampleTime=1.86011904761905e-08  RndMeth=Nearest
  Simple Dual Port RAM : hdlsllib/HDL RAMs/Simple Dual Port RAM  ram_size=9
      settings: SourceProductName=HDL Coder  SourceProductBaseCode=HD
  Sum : Sum  AccumDataTypeStr=fixdt(0, 11, 0)  OutDataTypeStr=fixdt(0, 9, 0)  SampleTime=1.86011904761905e-08
  Sum1 : Sum  AccumDataTypeStr=fixdt(0, 7, 0)  OutDataTypeStr=fixdt(0, 9, 0)  SampleTime=1.86011904761905e-08
  Switch : Switch  Criteria=u2 ~= 0  Threshold=double(0)  OutDataTypeStr=fixdt(0, 9, 0)  SampleTime=1.86011904761905e-08
  get_bit : Subsystem
  dout : Outport
  probe : Outport  Port=2
  wires:
  shift/1 -> Relational Operator/2
  raddr/1 -> Switch/3, Sum/2
  we/1 -> get_bit/1(u)
  waddr/1 -> Simple Dual Port RAM/2
  wdata/1 -> Simple Dual Port RAM/1
  i/1 -> Sum1/1, Relational Operator/1
  Constant/1 -> Sum/1
  Constant1/1 -> Sum1/2
  Relational Operator/1 -> Switch/2
  Simple Dual Port RAM/1 -> dout/1
  Sum/1 -> Switch/1
  Sum1/1 -> get_bit/2(ind)
  Switch/1 -> Simple Dual Port RAM/4, probe/1
  get_bit/1(y) -> Simple Dual Port RAM/3

== system gm_ZynqBF_2tx_fpga/channel_estimator/peakdetect_ch1/correlator1/rx_ram_q_instance56 ==
  i : Inport  OutDataTypeStr=fixdt(0, 6, 0)  PortDimensions=1  SampleTime=1.86011904761905e-08
  wdata : Inport  Port=2  OutDataTypeStr=fixdt(1, 16, 15)  PortDimensions=1  SampleTime=1.86011904761905e-08
  waddr : Inport  Port=3  OutDataTypeStr=fixdt(0, 9, 0)  PortDimensions=1  SampleTime=1.86011904761905e-08
  we : Inport  Port=4  OutDataTypeStr=fixdt(0, 64, 0)  PortDimensions=1  SampleTime=1.86011904761905e-08
  raddr : Inport  Port=5  OutDataTypeStr=fixdt(0, 10, 0)  PortDimensions=1  SampleTime=1.86011904761905e-08
  shift : Inport  Port=6  OutDataTypeStr=fixdt(0, 6, 0)  PortDimensions=1  SampleTime=1.86011904761905e-08
  Constant : Constant  OutDataTypeStr=fixdt(0, 1, 0)  SampleTime=-1
  Constant1 : Constant  OutDataTypeStr=fixdt(0, 1, 0)  SampleTime=-1
  Relational Operator : RelationalOperator  Operator=<  OutDataTypeStr=boolean  SampleTime=1.86011904761905e-08  RndMeth=Nearest
  Simple Dual Port RAM : hdlsllib/HDL RAMs/Simple Dual Port RAM  ram_size=9
      settings: SourceProductName=HDL Coder  SourceProductBaseCode=HD
  Sum : Sum  AccumDataTypeStr=fixdt(0, 11, 0)  OutDataTypeStr=fixdt(0, 9, 0)  SampleTime=1.86011904761905e-08
  Sum1 : Sum  AccumDataTypeStr=fixdt(0, 7, 0)  OutDataTypeStr=fixdt(0, 9, 0)  SampleTime=1.86011904761905e-08
  Switch : Switch  Criteria=u2 ~= 0  Threshold=double(0)  OutDataTypeStr=fixdt(0, 9, 0)  SampleTime=1.86011904761905e-08
  get_bit : Subsystem
  dout : Outport
  probe : Outport  Port=2
  wires:
  shift/1 -> Relational Operator/2
  raddr/1 -> Switch/3, Sum/2
  we/1 -> get_bit/1(u)
  waddr/1 -> Simple Dual Port RAM/2
  wdata/1 -> Simple Dual Port RAM/1
  i/1 -> Sum1/1, Relational Operator/1
  Constant/1 -> Sum/1
  Constant1/1 -> Sum1/2
  Relational Operator/1 -> Switch/2
  Simple Dual Port RAM/1 -> dout/1
  Sum/1 -> Switch/1
  Sum1/1 -> get_bit/2(ind)
  Switch/1 -> Simple Dual Port RAM/4, probe/1
  get_bit/1(y) -> Simple Dual Port RAM/3

== system gm_ZynqBF_2tx_fpga/channel_estimator/peakdetect_ch1/correlator1/rx_ram_q_instance57 ==
  i : Inport  OutDataTypeStr=fixdt(0, 6, 0)  PortDimensions=1  SampleTime=1.86011904761905e-08
  wdata : Inport  Port=2  OutDataTypeStr=fixdt(1, 16, 15)  PortDimensions=1  SampleTime=1.86011904761905e-08
  waddr : Inport  Port=3  OutDataTypeStr=fixdt(0, 9, 0)  PortDimensions=1  SampleTime=1.86011904761905e-08
  we : Inport  Port=4  OutDataTypeStr=fixdt(0, 64, 0)  PortDimensions=1  SampleTime=1.86011904761905e-08
  raddr : Inport  Port=5  OutDataTypeStr=fixdt(0, 10, 0)  PortDimensions=1  SampleTime=1.86011904761905e-08
  shift : Inport  Port=6  OutDataTypeStr=fixdt(0, 6, 0)  PortDimensions=1  SampleTime=1.86011904761905e-08
  Constant : Constant  OutDataTypeStr=fixdt(0, 1, 0)  SampleTime=-1
  Constant1 : Constant  OutDataTypeStr=fixdt(0, 1, 0)  SampleTime=-1
  Relational Operator : RelationalOperator  Operator=<  OutDataTypeStr=boolean  SampleTime=1.86011904761905e-08  RndMeth=Nearest
  Simple Dual Port RAM : hdlsllib/HDL RAMs/Simple Dual Port RAM  ram_size=9
      settings: SourceProductName=HDL Coder  SourceProductBaseCode=HD
  Sum : Sum  AccumDataTypeStr=fixdt(0, 11, 0)  OutDataTypeStr=fixdt(0, 9, 0)  SampleTime=1.86011904761905e-08
  Sum1 : Sum  AccumDataTypeStr=fixdt(0, 7, 0)  OutDataTypeStr=fixdt(0, 9, 0)  SampleTime=1.86011904761905e-08
  Switch : Switch  Criteria=u2 ~= 0  Threshold=double(0)  OutDataTypeStr=fixdt(0, 9, 0)  SampleTime=1.86011904761905e-08
  get_bit : Subsystem
  dout : Outport
  probe : Outport  Port=2
  wires:
  shift/1 -> Relational Operator/2
  raddr/1 -> Switch/3, Sum/2
  we/1 -> get_bit/1(u)
  waddr/1 -> Simple Dual Port RAM/2
  wdata/1 -> Simple Dual Port RAM/1
  i/1 -> Sum1/1, Relational Operator/1
  Constant/1 -> Sum/1
  Constant1/1 -> Sum1/2
  Relational Operator/1 -> Switch/2
  Simple Dual Port RAM/1 -> dout/1
  Sum/1 -> Switch/1
  Sum1/1 -> get_bit/2(ind)
  Switch/1 -> Simple Dual Port RAM/4, probe/1
  get_bit/1(y) -> Simple Dual Port RAM/3

== system gm_ZynqBF_2tx_fpga/channel_estimator/peakdetect_ch1/correlator1/rx_ram_q_instance58 ==
  i : Inport  OutDataTypeStr=fixdt(0, 6, 0)  PortDimensions=1  SampleTime=1.86011904761905e-08
  wdata : Inport  Port=2  OutDataTypeStr=fixdt(1, 16, 15)  PortDimensions=1  SampleTime=1.86011904761905e-08
  waddr : Inport  Port=3  OutDataTypeStr=fixdt(0, 9, 0)  PortDimensions=1  SampleTime=1.86011904761905e-08
  we : Inport  Port=4  OutDataTypeStr=fixdt(0, 64, 0)  PortDimensions=1  SampleTime=1.86011904761905e-08
  raddr : Inport  Port=5  OutDataTypeStr=fixdt(0, 10, 0)  PortDimensions=1  SampleTime=1.86011904761905e-08
  shift : Inport  Port=6  OutDataTypeStr=fixdt(0, 6, 0)  PortDimensions=1  SampleTime=1.86011904761905e-08
  Constant : Constant  OutDataTypeStr=fixdt(0, 1, 0)  SampleTime=-1
  Constant1 : Constant  OutDataTypeStr=fixdt(0, 1, 0)  SampleTime=-1
  Relational Operator : RelationalOperator  Operator=<  OutDataTypeStr=boolean  SampleTime=1.86011904761905e-08  RndMeth=Nearest
  Simple Dual Port RAM : hdlsllib/HDL RAMs/Simple Dual Port RAM  ram_size=9
      settings: SourceProductName=HDL Coder  SourceProductBaseCode=HD
  Sum : Sum  AccumDataTypeStr=fixdt(0, 11, 0)  OutDataTypeStr=fixdt(0, 9, 0)  SampleTime=1.86011904761905e-08
  Sum1 : Sum  AccumDataTypeStr=fixdt(0, 7, 0)  OutDataTypeStr=fixdt(0, 9, 0)  SampleTime=1.86011904761905e-08
  Switch : Switch  Criteria=u2 ~= 0  Threshold=double(0)  OutDataTypeStr=fixdt(0, 9, 0)  SampleTime=1.86011904761905e-08
  get_bit : Subsystem
  dout : Outport
  probe : Outport  Port=2
  wires:
  shift/1 -> Relational Operator/2
  raddr/1 -> Switch/3, Sum/2
  we/1 -> get_bit/1(u)
  waddr/1 -> Simple Dual Port RAM/2
  wdata/1 -> Simple Dual Port RAM/1
  i/1 -> Sum1/1, Relational Operator/1
  Constant/1 -> Sum/1
  Constant1/1 -> Sum1/2
  Relational Operator/1 -> Switch/2
  Simple Dual Port RAM/1 -> dout/1
  Sum/1 -> Switch/1
  Sum1/1 -> get_bit/2(ind)
  Switch/1 -> Simple Dual Port RAM/4, probe/1
  get_bit/1(y) -> Simple Dual Port RAM/3

== system gm_ZynqBF_2tx_fpga/channel_estimator/peakdetect_ch1/correlator1/rx_ram_q_instance59 ==
  i : Inport  OutDataTypeStr=fixdt(0, 6, 0)  PortDimensions=1  SampleTime=1.86011904761905e-08
  wdata : Inport  Port=2  OutDataTypeStr=fixdt(1, 16, 15)  PortDimensions=1  SampleTime=1.86011904761905e-08
  waddr : Inport  Port=3  OutDataTypeStr=fixdt(0, 9, 0)  PortDimensions=1  SampleTime=1.86011904761905e-08
  we : Inport  Port=4  OutDataTypeStr=fixdt(0, 64, 0)  PortDimensions=1  SampleTime=1.86011904761905e-08
  raddr : Inport  Port=5  OutDataTypeStr=fixdt(0, 10, 0)  PortDimensions=1  SampleTime=1.86011904761905e-08
  shift : Inport  Port=6  OutDataTypeStr=fixdt(0, 6, 0)  PortDimensions=1  SampleTime=1.86011904761905e-08
  Constant : Constant  OutDataTypeStr=fixdt(0, 1, 0)  SampleTime=-1
  Constant1 : Constant  OutDataTypeStr=fixdt(0, 1, 0)  SampleTime=-1
  Relational Operator : RelationalOperator  Operator=<  OutDataTypeStr=boolean  SampleTime=1.86011904761905e-08  RndMeth=Nearest
  Simple Dual Port RAM : hdlsllib/HDL RAMs/Simple Dual Port RAM  ram_size=9
      settings: SourceProductName=HDL Coder  SourceProductBaseCode=HD
  Sum : Sum  AccumDataTypeStr=fixdt(0, 11, 0)  OutDataTypeStr=fixdt(0, 9, 0)  SampleTime=1.86011904761905e-08
  Sum1 : Sum  AccumDataTypeStr=fixdt(0, 7, 0)  OutDataTypeStr=fixdt(0, 9, 0)  SampleTime=1.86011904761905e-08
  Switch : Switch  Criteria=u2 ~= 0  Threshold=double(0)  OutDataTypeStr=fixdt(0, 9, 0)  SampleTime=1.86011904761905e-08
  get_bit : Subsystem
  dout : Outport
  probe : Outport  Port=2
  wires:
  shift/1 -> Relational Operator/2
  raddr/1 -> Switch/3, Sum/2
  we/1 -> get_bit/1(u)
  waddr/1 -> Simple Dual Port RAM/2
  wdata/1 -> Simple Dual Port RAM/1
  i/1 -> Sum1/1, Relational Operator/1
  Constant/1 -> Sum/1
  Constant1/1 -> Sum1/2
  Relational Operator/1 -> Switch/2
  Simple Dual Port RAM/1 -> dout/1
  Sum/1 -> Switch/1
  Sum1/1 -> get_bit/2(ind)
  Switch/1 -> Simple Dual Port RAM/4, probe/1
  get_bit/1(y) -> Simple Dual Port RAM/3

== system gm_ZynqBF_2tx_fpga/channel_estimator/peakdetect_ch1/correlator1/rx_ram_q_instance6 ==
  i : Inport  OutDataTypeStr=fixdt(0, 6, 0)  PortDimensions=1  SampleTime=1.86011904761905e-08
  wdata : Inport  Port=2  OutDataTypeStr=fixdt(1, 16, 15)  PortDimensions=1  SampleTime=1.86011904761905e-08
  waddr : Inport  Port=3  OutDataTypeStr=fixdt(0, 9, 0)  PortDimensions=1  SampleTime=1.86011904761905e-08
  we : Inport  Port=4  OutDataTypeStr=fixdt(0, 64, 0)  PortDimensions=1  SampleTime=1.86011904761905e-08
  raddr : Inport  Port=5  OutDataTypeStr=fixdt(0, 10, 0)  PortDimensions=1  SampleTime=1.86011904761905e-08
  shift : Inport  Port=6  OutDataTypeStr=fixdt(0, 6, 0)  PortDimensions=1  SampleTime=1.86011904761905e-08
  Constant : Constant  OutDataTypeStr=fixdt(0, 1, 0)  SampleTime=-1
  Constant1 : Constant  OutDataTypeStr=fixdt(0, 1, 0)  SampleTime=-1
  Relational Operator : RelationalOperator  Operator=<  OutDataTypeStr=boolean  SampleTime=1.86011904761905e-08  RndMeth=Nearest
  Simple Dual Port RAM : hdlsllib/HDL RAMs/Simple Dual Port RAM  ram_size=9
      settings: SourceProductName=HDL Coder  SourceProductBaseCode=HD
  Sum : Sum  AccumDataTypeStr=fixdt(0, 11, 0)  OutDataTypeStr=fixdt(0, 9, 0)  SampleTime=1.86011904761905e-08
  Sum1 : Sum  AccumDataTypeStr=fixdt(0, 7, 0)  OutDataTypeStr=fixdt(0, 9, 0)  SampleTime=1.86011904761905e-08
  Switch : Switch  Criteria=u2 ~= 0  Threshold=double(0)  OutDataTypeStr=fixdt(0, 9, 0)  SampleTime=1.86011904761905e-08
  get_bit : Subsystem
  dout : Outport
  probe : Outport  Port=2
  wires:
  shift/1 -> Relational Operator/2
  raddr/1 -> Switch/3, Sum/2
  we/1 -> get_bit/1(u)
  waddr/1 -> Simple Dual Port RAM/2
  wdata/1 -> Simple Dual Port RAM/1
  i/1 -> Sum1/1, Relational Operator/1
  Constant/1 -> Sum/1
  Constant1/1 -> Sum1/2
  Relational Operator/1 -> Switch/2
  Simple Dual Port RAM/1 -> dout/1
  Sum/1 -> Switch/1
  Sum1/1 -> get_bit/2(ind)
  Switch/1 -> Simple Dual Port RAM/4, probe/1
  get_bit/1(y) -> Simple Dual Port RAM/3
